simulink model "L22"  (R2015a)
settings: Solver=ode45  StartTime=0.0  StopTime=1  MaxStep=1e-4  RelTol=1e-3
values from neighbouring files (symbols this model uses):
  a1 = ke*km/J/La    (= 10740.9160847)    [L22m.m]
  a2 = Ra/La    (= 294.117647059)    [L22m.m]
  alfaConstant = 1.31    [L22m.m]
  b = -km*kp/J/La    (= -1139188.06959)    [L22m.m]
  bB3 = 1138537    [L22m.m]
  c = 10000    [L22m.m]
  cB1 = 290    [L22m.m]
  deltaB2 = 0.2    [L22m.m]
  fi1 = -294.11    [L22m.m]
  fi2 = -10740    [L22m.m]
  fmaxB1 = 1e+7    (= 10000000)    [L22m.m]
  fmaxB2 = 1e+7    (= 10000000)    [L22m.m]
  J = 0.71e-3    (= 0.00071)    [L22m.m]
  kB3 = 5*1e+7    (= 50000000)    [L22m.m]
  ke = 0.33    [L22m.m]
  km = ke    (= 0.33)    [L22m.m]
  kp = 35    [L22m.m]
  kr = 1.1792    [L22m.m]
  La = 14.28e-3    (= 0.01428)    [L22m.m]
  Ra = 4.2    [L22m.m]
  Ti = 0.0234    [L22m.m]
  TiB1 = 0.0234    [L22m.m]
  v = -12    [L22m.m]
  vTime = 0.6    [L22m.m]
  w = 20    [L22m.m]
settings Model: Creator=B014-5  LastModifiedBy=B014-5

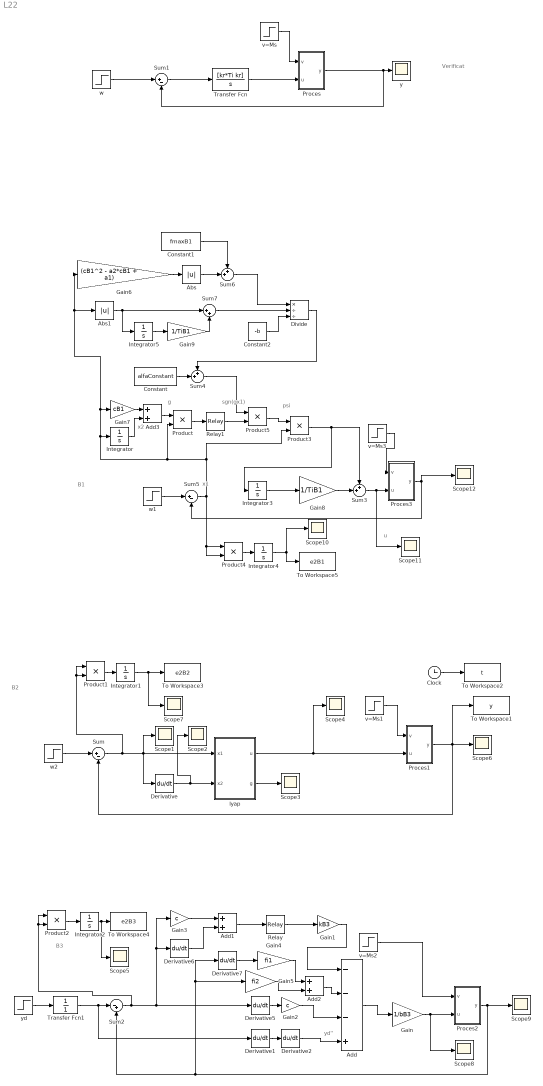
== system L22 ==
  note: Verificat
  note: B2
  note: yd''
  note: B3
  note: u
  note: psi
  note: g
  note: sgn(gx1)
  note: x2
  note: x1
  note: B1
  Abs : Abs
  Abs1 : Abs
  Add : Sum  Inputs=---+
  Add1 : Sum
  Add2 : Sum
  Add3 : Sum
  Clock : Clock
  Constant : Constant  Value=alfaConstant
  Constant1 : Constant  Value=fmaxB1
  Constant2 : Constant  Value=-b
  Derivative : Derivative
  Derivative{1..2,5..7} (5 alike) : Derivative  CoefficientInTFapproximation=1e+5
  Divide : Product  Inputs=*//
  Gain : Gain  Gain=1/bB3
  Gain1 : Gain  Gain=kB3
  Gain2 : Gain  Gain=c
  Gain3 : Gain  Gain=c
  Gain4 : Gain  Gain=fi1
  Gain5 : Gain  Gain=fi2
  Gain6 : Gain  Gain=(cB1^2 - a2*cB1 + a1)
  Gain7 : Gain  Gain=cB1
  Gain8 : Gain  Gain=1/TiB1
  Gain9 : Gain  Gain=1/TiB1
  Integrator{,1..5} (6 alike) : Integrator
  Proces : Subsystem
  Proces1 : Subsystem
  Proces2 : Subsystem
  Proces3 : Subsystem
  Product{,1..5} (6 alike) : Product
  Relay : Relay  OnSwitchValue=0  OffSwitchValue=0  OffOutputValue=-1  ZeroCross=off
  Relay1 : Relay  OnSwitchValue=0  OffSwitchValue=0  OffOutputValue=-1  ZeroCross=off
  Scope{1..12} (12 alike) : Scope
      Scope1 settings: SaveName=ScopeData7
      Scope11 settings: YMin=-4.25e+105  YMax=0  SaveName=ScopeData11
      Scope12 settings: YMin=-4.25e+105  YMax=0  SaveName=ScopeData12
      Scope2 settings: SaveName=ScopeData2
      Scope3 settings: SaveName=ScopeData3
      Scope4 settings: SaveName=ScopeData4
      Scope5 settings: SaveName=ScopeData9
      Scope6 settings: YMin=0  YMax=21  SaveName=ScopeData5
      Scope7 settings: SaveName=ScopeData8
      Scope8 settings: YMin=-4.25e+105  YMax=0  SaveName=ScopeData10
      Scope9 settings: YMin=-4.25e+105  YMax=0  SaveName=ScopeData6
  Sum : Sum  Inputs=|+-
  Sum1 : Sum  Inputs=|+-
  Sum2 : Sum  Inputs=|-+
  Sum3 : Sum  Inputs=++|
  Sum4 : Sum  Inputs=++|
  Sum5 : Sum  Inputs=|+-
  Sum6 : Sum  Inputs=++|
  Sum7 : Sum  Inputs=|++
  To Workspace1 : ToWorkspace  VariableName=y  SampleTime=-1
  To Workspace2 : ToWorkspace  VariableName=t  SampleTime=-1
  To Workspace3 : ToWorkspace  VariableName=e2B2  SampleTime=-1
  To Workspace4 : ToWorkspace  VariableName=e2B3  SampleTime=-1
  To Workspace5 : ToWorkspace  VariableName=e2B1  SampleTime=-1
  Transfer Fcn : TransferFcn  Numerator=[kr*Ti kr]  Denominator=[1 0]
  Transfer Fcn1 : TransferFcn  Denominator=[0.0 1]
  lyap : Subsystem
  v=Ms{,1..3} (4 alike) : Step  Time=vTime  After=v  SampleTime=0
  w : Step  Time=0  After=w  SampleTime=0
  w1 : Step  Time=0  After=w  SampleTime=0
  w2 : Step  Time=0  After=w  SampleTime=0
  y : Scope
  yd : Step  Time=0  After=w  SampleTime=0
  wires:
  v=Ms/1 -> Proces/1(v)
  Proces/1(y) -> Sum1/2, y/1
  w/1 -> Sum1/1
  Transfer Fcn/1 -> Proces/2(u)
  Sum1/1 -> Transfer Fcn/1
  w2/1 -> Sum/1
  Sum/1 -> Product1/1, Product1/2, Derivative/1, lyap/1(x1), Scope1/1
  Derivative/1 -> Scope2/1, lyap/2(x2)
  lyap/2(g) -> Scope3/1
  lyap/1(u) -> Proces1/2(u), Scope4/1
  v=Ms1/1 -> Proces1/1(v)
  Proces1/1(y) -> To Workspace1/1, Sum/2, Scope6/1
  Clock/1 -> To Workspace2/1
  Product1/1 -> Integrator1/1
  Integrator1/1 -> Scope7/1, To Workspace3/1
  Derivative1/1 -> Derivative2/1
  Proces2/1(y) -> Scope9/1, Sum2/2, Gain5/1, Derivative7/1
  Derivative5/1 -> Gain2/1
  v=Ms2/1 -> Proces2/1(v)
  Add/1 -> Gain/1
  Gain2/1 -> Add/3
  Add1/1 -> Relay/1
  Derivative6/1 -> Add1/2
  Gain3/1 -> Add1/1
  Relay/1 -> Gain1/1
  Gain1/1 -> Add/1
  Derivative7/1 -> Gain4/1
  Gain/1 -> Scope8/1, Proces2/2(u)
  Sum2/1 -> Gain3/1, Derivative6/1, Derivative5/1, Product2/1, Product2/2
  Product2/1 -> Integrator2/1
  Integrator2/1 -> Scope5/1, To Workspace4/1
  Derivative2/1 -> Add/4
  Add2/1 -> Add/2
  Gain4/1 -> Add2/1
  Gain5/1 -> Add2/2
  yd/1 -> Transfer Fcn1/1
  Transfer Fcn1/1 -> Derivative1/1, Sum2/1
  w1/1 -> Sum5/1
  Proces3/1(y) -> Sum5/2, Scope12/1
  Product3/1 -> Sum3/1, Integrator3/1
  Sum3/1 -> Proces3/2(u), Scope11/1
  Relay1/1 -> Product5/2
  Sum5/1 -> Product4/2, Product4/1, Product3/2, Product/2, Gain7/1, Abs1/1, Gain6/1, Integrator/1
  Gain7/1 -> Add3/1
  Integrator/1 -> Add3/2
  Product/1 -> Relay1/1
  Add3/1 -> Product/1
  Product5/1 -> Product3/1
  Integrator3/1 -> Gain8/1
  Gain8/1 -> Sum3/2
  v=Ms3/1 -> Proces3/1(v)
  Product4/1 -> Integrator4/1
  Integrator4/1 -> To Workspace5/1, Scope10/1
  Sum4/1 -> Product5/1
  Constant/1 -> Sum4/2
  Gain6/1 -> Abs/1
  Abs/1 -> Sum6/2
  Constant1/1 -> Sum6/1
  Sum6/1 -> Divide/1
  Abs1/1 -> Sum7/1, Integrator5/1
  Integrator5/1 -> Gain9/1
  Gain9/1 -> Sum7/2
  Sum7/1 -> Divide/2
  Divide/1 -> Sum4/1
  Constant2/1 -> Divide/3

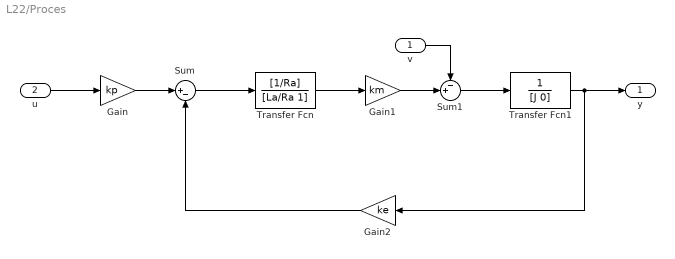
== system L22/Proces ==
  v : Inport
  u : Inport  Port=2
  Gain : Gain  Gain=kp
  Gain1 : Gain  Gain=km
  Gain2 : Gain  Gain=ke
  Sum : Sum  Inputs=|+-
  Sum1 : Sum  Inputs=-+|
  Transfer Fcn : TransferFcn  Numerator=[1/Ra]  Denominator=[La/Ra 1]
  Transfer Fcn1 : TransferFcn  Denominator=[J 0]
  y : Outport
  wires:
  v/1 -> Sum1/1
  Gain/1 -> Sum/1
  Transfer Fcn1/1 -> y/1, Gain2/1
  Sum1/1 -> Transfer Fcn1/1
  Sum/1 -> Transfer Fcn/1
  Gain2/1 -> Sum/2
  u/1 -> Gain/1
  Gain1/1 -> Sum1/2
  Transfer Fcn/1 -> Gain1/1

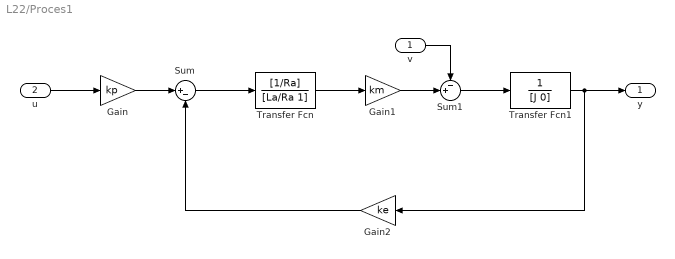
== system L22/Proces1 ==
  v : Inport
  u : Inport  Port=2
  Gain : Gain  Gain=kp
  Gain1 : Gain  Gain=km
  Gain2 : Gain  Gain=ke
  Sum : Sum  Inputs=|+-
  Sum1 : Sum  Inputs=-+|
  Transfer Fcn : TransferFcn  Numerator=[1/Ra]  Denominator=[La/Ra 1]
  Transfer Fcn1 : TransferFcn  Denominator=[J 0]
  y : Outport
  wires:
  v/1 -> Sum1/1
  Gain/1 -> Sum/1
  Transfer Fcn1/1 -> y/1, Gain2/1
  Sum1/1 -> Transfer Fcn1/1
  Sum/1 -> Transfer Fcn/1
  Gain2/1 -> Sum/2
  u/1 -> Gain/1
  Gain1/1 -> Sum1/2
  Transfer Fcn/1 -> Gain1/1

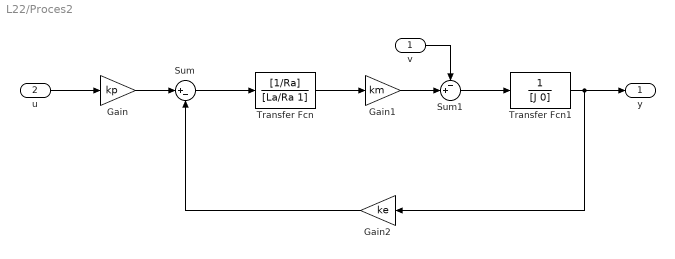
== system L22/Proces2 ==
  v : Inport
  u : Inport  Port=2
  Gain : Gain  Gain=kp
  Gain1 : Gain  Gain=km
  Gain2 : Gain  Gain=ke
  Sum : Sum  Inputs=|+-
  Sum1 : Sum  Inputs=-+|
  Transfer Fcn : TransferFcn  Numerator=[1/Ra]  Denominator=[La/Ra 1]
  Transfer Fcn1 : TransferFcn  Denominator=[J 0]
  y : Outport
  wires:
  Transfer Fcn/1 -> Gain1/1
  Gain1/1 -> Sum1/2
  u/1 -> Gain/1
  Gain2/1 -> Sum/2
  Sum/1 -> Transfer Fcn/1
  Sum1/1 -> Transfer Fcn1/1
  Transfer Fcn1/1 -> Gain2/1, y/1
  Gain/1 -> Sum/1
  v/1 -> Sum1/1

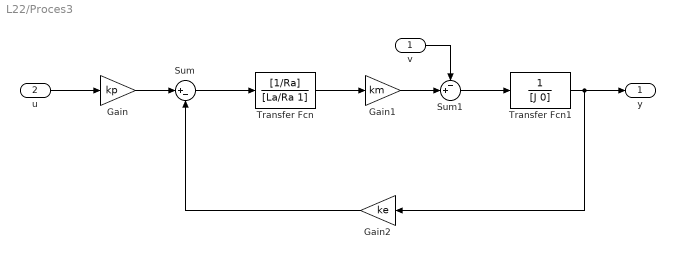
== system L22/Proces3 ==
  v : Inport
  u : Inport  Port=2
  Gain : Gain  Gain=kp
  Gain1 : Gain  Gain=km
  Gain2 : Gain  Gain=ke
  Sum : Sum  Inputs=|+-
  Sum1 : Sum  Inputs=-+|
  Transfer Fcn : TransferFcn  Numerator=[1/Ra]  Denominator=[La/Ra 1]
  Transfer Fcn1 : TransferFcn  Denominator=[J 0]
  y : Outport
  wires:
  v/1 -> Sum1/1
  Gain/1 -> Sum/1
  Transfer Fcn1/1 -> y/1, Gain2/1
  Sum1/1 -> Transfer Fcn1/1
  Sum/1 -> Transfer Fcn/1
  Gain2/1 -> Sum/2
  u/1 -> Gain/1
  Gain1/1 -> Sum1/2
  Transfer Fcn/1 -> Gain1/1

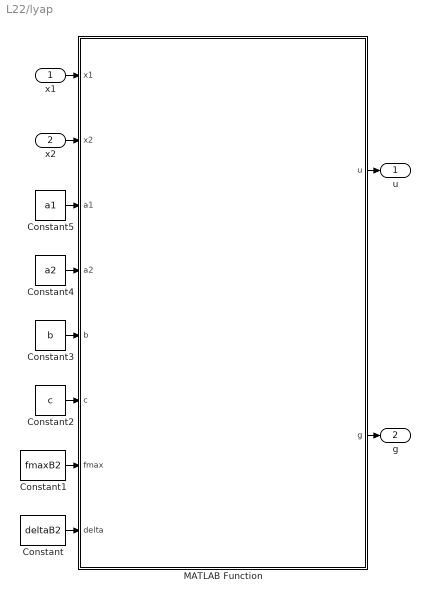
== system L22/lyap ==
  x1 : Inport
  x2 : Inport  Port=2
  Constant : Constant  Value=deltaB2
  Constant1 : Constant  Value=fmaxB2
  Constant2 : Constant  Value=c
  Constant3 : Constant  Value=b
  Constant4 : Constant  Value=a2
  Constant5 : Constant  Value=a1
  MATLAB Function : MATLAB Function  TreatAsAtomicUnit=on
  u : Outport
  g : Outport  Port=2
  wires:
  Constant2/1 -> MATLAB Function/6(c)
  Constant5/1 -> MATLAB Function/3(a1)
  Constant1/1 -> MATLAB Function/7(fmax)
  Constant4/1 -> MATLAB Function/4(a2)
  x2/1 -> MATLAB Function/2(x2)
  MATLAB Function/2(g) -> g/1
  Constant/1 -> MATLAB Function/8(delta)
  MATLAB Function/1(u) -> u/1
  x1/1 -> MATLAB Function/1(x1)
  Constant3/1 -> MATLAB Function/5(b)

== matlab function L22/lyap/MATLAB Function ==
  data: u output; g output; x1 input; x2 input; a1 input; a2 input; b input; c input; fmax input; delta input
function [u, g] = lyap(x1, x2, a1, a2, b, c, fmax, delta)
%#codegen

g = c * x1 + x2;
u = sign(g)*(abs((a1*x1-(c-a2)*x2)+fmax)/abs(b)+delta);
